simulink model "Demo_SteerableHeadlights_cs"  (R2014b)
settings: Solver=FixedStepDiscrete  SolverMode=SingleTasking  StartTime=0.0  StopTime=45  FixedStep=1/20  RelTol=1e-3
PreLoadFcn:
  | mbxruntime.callbacks.PreLoadFcn(bdroot);
  | check_NUTS_defined;
  | 
  | assignin('base',['model_closed_' bdroot],false);
PostLoadFcn:
  | mbxruntime.callbacks.PostLoadFcn(bdroot);
InitFcn:
  | mbxruntime.callbacks.InitFcn(bdroot);
StartFcn:
  | mbxruntime.callbacks.StartFcn(bdroot);
  | 
  | open_system([bdroot '/BMW_X5_1/Scope: steer angle, preview angle, selected angle']);
StopFcn:
  | mbxruntime.callbacks.StopFcn(bdroot);
model workspace: external: MAT-File .\Demo_SteerableHeadlights_cs_hws.mat (data not in the file)
undefined symbols (not defined in the file or in its folder): mbxruntime, tabledata
undefined symbols (not defined in the file): Demo_SteerableHeadlights_cs_1a268cb91cfaa718, Demo_SteerableHeadlights_cs_a8b5e2ccc8aad9ca, Demo_SteerableHeadlights_cs_BMW_X5_1_Path_pathUniqueID, Demo_SteerableHeadlights_cs_HumanTextured_1_Path_pathUniqueID, SteeringColumn, SteeringWheel, WheelL0, WheelL1, WheelR0, WheelR1
libraries: simulink_extras x15, simulink x2
(part 2 of 5)

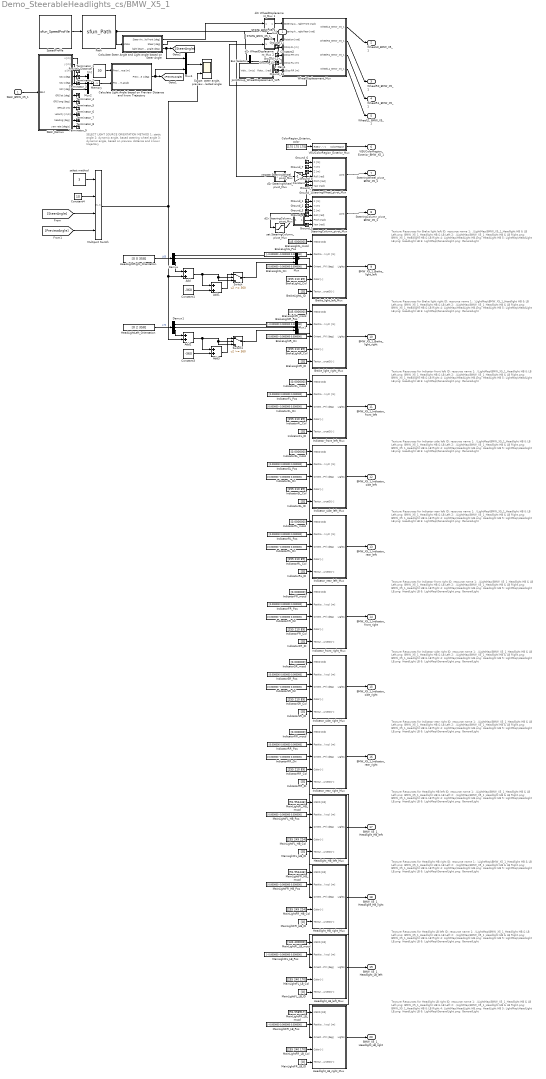
== system Demo_SteerableHeadlights_cs/BMW_X5_1 ==
  note: Texture Resources for Brake light left
      |
      | ID: resource name
      | 1: .\LightMap\BMW_X5_1_Headlight HB & LB Left.png: BMW_X5_1_Headlight HB & LB Left
      | 2: .\LightMap\BMW_X5_1_Headlight HB & LB Right.png: BMW_X5_1_Headlight HB & LB Right
      | 4: LightMap\HeadLight HB.png: HeadLight HB
      | 5: LightMap\HeadLight LB.png: HeadLight LB
      | 6: LightMap\GeneralLight.png: GeneralLight
  note: Texture Resources for Brake light right
      |
      | ID: resource name
      | 1: .\LightMap\BMW_X5_1_Headlight HB & LB Left.png: BMW_X5_1_Headlight HB & LB Left
      | 2: .\LightMap\BMW_X5_1_Headlight HB & LB Right.png: BMW_X5_1_Headlight HB & LB Right
      | 4: LightMap\HeadLight HB.png: HeadLight HB
      | 5: LightMap\HeadLight LB.png: HeadLight LB
      | 6: LightMap\GeneralLight.png: GeneralLight
  note: Texture Resources for Indicator front left
      |
      | ID: resource name
      | 1: .\LightMap\BMW_X5_1_Headlight HB & LB Left.png: BMW_X5_1_Headlight HB & LB Left
      | 2: .\LightMap\BMW_X5_1_Headlight HB & LB Right.png: BMW_X5_1_Headlight HB & LB Right
      | 4: LightMap\HeadLight HB.png: HeadLight HB
      | 5: LightMap\HeadLight LB.png: HeadLight LB
      | 6: LightMap\GeneralLight.png: GeneralLight
  note: Texture Resources for Indicator side left
      |
      | ID: resource name
      | 1: .\LightMap\BMW_X5_1_Headlight HB & LB Left.png: BMW_X5_1_Headlight HB & LB Left
      | 2: .\LightMap\BMW_X5_1_Headlight HB & LB Right.png: BMW_X5_1_Headlight HB & LB Right
      | 4: LightMap\HeadLight HB.png: HeadLight HB
      | 5: LightMap\HeadLight LB.png: HeadLight LB
      | 6: LightMap\GeneralLight.png: GeneralLight
  note: Texture Resources for Indicator rear left
      |
      | ID: resource name
      | 1: .\LightMap\BMW_X5_1_Headlight HB & LB Left.png: BMW_X5_1_Headlight HB & LB Left
      | 2: .\LightMap\BMW_X5_1_Headlight HB & LB Right.png: BMW_X5_1_Headlight HB & LB Right
      | 4: LightMap\HeadLight HB.png: HeadLight HB
      | 5: LightMap\HeadLight LB.png: HeadLight LB
      | 6: LightMap\GeneralLight.png: GeneralLight
  note: Texture Resources for Indicator front right
      |
      | ID: resource name
      | 1: .\LightMap\BMW_X5_1_Headlight HB & LB Left.png: BMW_X5_1_Headlight HB & LB Left
      | 2: .\LightMap\BMW_X5_1_Headlight HB & LB Right.png: BMW_X5_1_Headlight HB & LB Right
      | 4: LightMap\HeadLight HB.png: HeadLight HB
      | 5: LightMap\HeadLight LB.png: HeadLight LB
      | 6: LightMap\GeneralLight.png: GeneralLight
  note: Texture Resources for Indicator side right
      |
      | ID: resource name
      | 1: .\LightMap\BMW_X5_1_Headlight HB & LB Left.png: BMW_X5_1_Headlight HB & LB Left
      | 2: .\LightMap\BMW_X5_1_Headlight HB & LB Right.png: BMW_X5_1_Headlight HB & LB Right
      | 4: LightMap\HeadLight HB.png: HeadLight HB
      | 5: LightMap\HeadLight LB.png: HeadLight LB
      | 6: LightMap\GeneralLight.png: GeneralLight
  note: Texture Resources for Indicator rear right
      |
      | ID: resource name
      | 1: .\LightMap\BMW_X5_1_Headlight HB & LB Left.png: BMW_X5_1_Headlight HB & LB Left
      | 2: .\LightMap\BMW_X5_1_Headlight HB & LB Right.png: BMW_X5_1_Headlight HB & LB Right
      | 4: LightMap\HeadLight HB.png: HeadLight HB
      | 5: LightMap\HeadLight LB.png: HeadLight LB
      | 6: LightMap\GeneralLight.png: GeneralLight
  note: Texture Resources for Headlight HB left
      |
      | ID: resource name
      | 1: .\LightMap\BMW_X5_1_Headlight HB & LB Left.png: BMW_X5_1_Headlight HB & LB Left
      | 2: .\LightMap\BMW_X5_1_Headlight HB & LB Right.png: BMW_X5_1_Headlight HB & LB Right
      | 4: LightMap\HeadLight HB.png: HeadLight HB
      | 5: LightMap\HeadLight LB.png: HeadLight LB
      | 6: LightMap\GeneralLight.png: GeneralLight
  note: Texture Resources for Headlight HB right
      |
      | ID: resource name
      | 1: .\LightMap\BMW_X5_1_Headlight HB & LB Left.png: BMW_X5_1_Headlight HB & LB Left
      | 2: .\LightMap\BMW_X5_1_Headlight HB & LB Right.png: BMW_X5_1_Headlight HB & LB Right
      | 4: LightMap\HeadLight HB.png: HeadLight HB
      | 5: LightMap\HeadLight LB.png: HeadLight LB
      | 6: LightMap\GeneralLight.png: GeneralLight
  note: Texture Resources for Headlight LB left
      |
      | ID: resource name
      | 1: .\LightMap\BMW_X5_1_Headlight HB & LB Left.png: BMW_X5_1_Headlight HB & LB Left
      | 2: .\LightMap\BMW_X5_1_Headlight HB & LB Right.png: BMW_X5_1_Headlight HB & LB Right
      | 4: LightMap\HeadLight HB.png: HeadLight HB
      | 5: LightMap\HeadLight LB.png: HeadLight LB
      | 6: LightMap\GeneralLight.png: GeneralLight
  note: Texture Resources for Headlight LB right
      |
      | ID: resource name
      | 1: .\LightMap\BMW_X5_1_Headlight HB & LB Left.png: BMW_X5_1_Headlight HB & LB Left
      | 2: .\LightMap\BMW_X5_1_Headlight HB & LB Right.png: BMW_X5_1_Headlight HB & LB Right
      | 4: LightMap\HeadLight HB.png: HeadLight HB
      | 5: LightMap\HeadLight LB.png: HeadLight LB
      | 6: LightMap\GeneralLight.png: GeneralLight
  note: SELECT LIGHT SOURCE ORIENTATION METHOD
      | 1: static angle
      | 2: dynamic angle, based steering wheel angle
      | 3: dynamic angle, based on preview distance
      |     and known trajectory
  SELF_BMW_X5_1 : Inport  Tag=inport/SelfPort  OutDataTypeStr=Bus: PRESCAN_SELFSENSORDATA  PortDimensions=1  SampleTime=1/20  BusOutputAsStruct=on
  Add{,1..3} (4 alike) : Sum
  BrakeLightL_Col : Constant  Tag=VisuLightConst  Value=[255 210 89]
  BrakeLightL_ID : Constant  Tag=VisuLightConst  Value=[0]
  BrakeLightL_Ori : Constant  Tag=VisuLightConst  Value=[0.000000 -0.000000 0.000000]
  BrakeLightL_Pos : Constant  Tag=VisuLightConst  Value=[-0.000000 -0.000000 0.000000]
  BrakeLightL_mscd : Constant  Tag=VisuLightConst  Value=[45.000000]
  BrakeLightR_Col : Constant  Tag=VisuLightConst  Value=[255 210 89]
  BrakeLightR_ID : Constant  Tag=VisuLightConst  Value=[0]
  BrakeLightR_Ori : Constant  Tag=VisuLightConst  Value=[0.000000 -0.000000 0.000000]
  BrakeLightR_Pos : Constant  Tag=VisuLightConst  Value=[-0.000000 0.000000 0.000000]
  BrakeLightR_mscd : Constant  Tag=VisuLightConst  Value=[45.000000]
  Brake_light_left_Mux : Subsystem  Tag=mux/ActiveLight  mask(PreScan User Interface: VisuActiveLight){}
      mask help:
      | The VisuActiveLight block provides a way for detailed animation of Light Sources, such as the indicator, brake, fog and main lights of a vehicle, or a light post.
      |
      | For more information, please click Help.
      settings: DeleteFcn=PreScanBlockDeleteFcn;
      mask Help: eval('openHelp(209)')
  Brake_light_right_Mux : Subsystem  Tag=mux/ActiveLight  mask(PreScan User Interface: VisuActiveLight){}
      mask help:
      | The VisuActiveLight block provides a way for detailed animation of Light Sources, such as the indicator, brake, fog and main lights of a vehicle, or a light post.
      |
      | For more information, please click Help.
      settings: DeleteFcn=PreScanBlockDeleteFcn;
      mask Help: eval('openHelp(209)')
  Bus Selector : BusSelector  OutputSignals=VelocityX
  Calculate Light Angle based on Preview Distance and know Trajectory : Subsystem  mask{FileName=PathFollowerSva_1_Synced.mat, TrajOffset=[0 0 0]}
      mask prompts: FileName "Trajectory Name"; TrajOffset "Trajectory Initial Offset x,y,yawangle [m,m,rad]"
      mask init:
      | load(['Trajectories/',FileName])
      | traject=trajectory';
      | 
      | 
      | Traj_x=(traject(:,2)*cos(TrajOffset(3))-traject(:,3)*sin(TrajOffset(3)))+TrajOffset(1);
      | Traj_y=(traject(:,2)*sin(TrajOffset(3))+traject(:,3)*cos(TrajOffset(3)))+TrajOffset(2);
  Calculate Steer Angle and Light angle based on Steer Angle : Subsystem
  ColorRegion_Exterior_color : Constant  Tag=VisuLightConst  Value=[175 175 175]
  Constant : Constant  Value=17
  Constant1 : Constant  Value=-360
  Constant2 : Constant  Value=0
  Constant3 : Constant  Value=-360
  Constant4 : Constant  Value=10
  Demux : Demux  Outputs=3
  Demux1 : Demux  Outputs=3
  Gain4 : Gain  Gain=-1*1.2
  Ground_{1..14} (14 alike) : Ground
  HeadLightLeft_Orientation : Constant  Value=[0 2 358]
  HeadLightRight_Orientation : Constant  Value=[0 0 358]
  Headlight_HB_left_Mux : Subsystem  Tag=mux/ActiveLight  mask(PreScan User Interface: VisuActiveLight){}
      mask help:
      | The VisuActiveLight block provides a way for detailed animation of Light Sources, such as the indicator, brake, fog and main lights of a vehicle, or a light post.
      |
      | For more information, please click Help.
      settings: DeleteFcn=PreScanBlockDeleteFcn;
      mask Help: eval('openHelp(209)')
  Headlight_HB_right_Mux : Subsystem  Tag=mux/ActiveLight  mask(PreScan User Interface: VisuActiveLight){}
      mask help:
      | The VisuActiveLight block provides a way for detailed animation of Light Sources, such as the indicator, brake, fog and main lights of a vehicle, or a light post.
      |
      | For more information, please click Help.
      settings: DeleteFcn=PreScanBlockDeleteFcn;
      mask Help: eval('openHelp(209)')
  Headlight_LB_left_Mux : Subsystem  Tag=mux/ActiveLight  mask(PreScan User Interface: VisuActiveLight){}
      mask help:
      | The VisuActiveLight block provides a way for detailed animation of Light Sources, such as the indicator, brake, fog and main lights of a vehicle, or a light post.
      |
      | For more information, please click Help.
      settings: DeleteFcn=PreScanBlockDeleteFcn;
      mask Help: eval('openHelp(209)')
  Headlight_LB_right_Mux : Subsystem  Tag=mux/ActiveLight  mask(PreScan User Interface: VisuActiveLight){}
      mask help:
      | The VisuActiveLight block provides a way for detailed animation of Light Sources, such as the indicator, brake, fog and main lights of a vehicle, or a light post.
      |
      | For more information, please click Help.
      settings: DeleteFcn=PreScanBlockDeleteFcn;
      mask Help: eval('openHelp(209)')
  IndicatorFL_Col : Constant  Tag=VisuLightConst  Value=[255 210 89]
  IndicatorFL_ID : Constant  Tag=VisuLightConst  Value=[0]
  IndicatorFL_Ori : Constant  Tag=VisuLightConst  Value=[0.000000 -0.000000 0.000000]
  IndicatorFL_Pos : Constant  Tag=VisuLightConst  Value=[0.000000 0.000000 0.000000]
  IndicatorFL_mscd : Constant  Tag=VisuLightConst  Value=[0.000000]
  IndicatorFR_Col : Constant  Tag=VisuLightConst  Value=[255 210 89]
  IndicatorFR_ID : Constant  Tag=VisuLightConst  Value=[0]
  IndicatorFR_Ori : Constant  Tag=VisuLightConst  Value=[0.000000 -0.000000 0.000000]
  IndicatorFR_Pos : Constant  Tag=VisuLightConst  Value=[0.000000 0.000000 0.000000]
  IndicatorFR_mscd : Constant  Tag=VisuLightConst  Value=[0.000000]
  IndicatorRL_Col : Constant  Tag=VisuLightConst  Value=[255 210 89]
  IndicatorRL_ID : Constant  Tag=VisuLightConst  Value=[0]
  IndicatorRL_Ori : Constant  Tag=VisuLightConst  Value=[0.000000 -0.000000 0.000000]
  IndicatorRL_Pos : Constant  Tag=VisuLightConst  Value=[0.000000 0.000000 0.000000]
  IndicatorRL_mscd : Constant  Tag=VisuLightConst  Value=[0.000000]
  IndicatorRR_Col : Constant  Tag=VisuLightConst  Value=[255 210 89]
  IndicatorRR_ID : Constant  Tag=VisuLightConst  Value=[0]
  IndicatorRR_Ori : Constant  Tag=VisuLightConst  Value=[0.000000 -0.000000 0.000000]
  IndicatorRR_Pos : Constant  Tag=VisuLightConst  Value=[0.000000 0.000000 0.000000]
  IndicatorRR_mscd : Constant  Tag=VisuLightConst  Value=[0.000000]
  IndicatorSL_Col : Constant  Tag=VisuLightConst  Value=[255 210 89]
  IndicatorSL_ID : Constant  Tag=VisuLightConst  Value=[0]
  IndicatorSL_Ori : Constant  Tag=VisuLightConst  Value=[0.000000 -0.000000 0.000000]
  IndicatorSL_Pos : Constant  Tag=VisuLightConst  Value=[0.000000 0.000000 0.000000]
  IndicatorSL_mscd : Constant  Tag=VisuLightConst  Value=[0.000000]
  IndicatorSR_Col : Constant  Tag=VisuLightConst  Value=[255 210 89]
  IndicatorSR_ID : Constant  Tag=VisuLightConst  Value=[0]
  IndicatorSR_Ori : Constant  Tag=VisuLightConst  Value=[0.000000 -0.000000 0.000000]
  IndicatorSR_Pos : Constant  Tag=VisuLightConst  Value=[0.000000 0.000000 0.000000]
  IndicatorSR_mscd : Constant  Tag=VisuLightConst  Value=[0.000000]
  Indicator_front_left_Mux : Subsystem  Tag=mux/ActiveLight  mask(PreScan User Interface: VisuActiveLight){}
      mask help:
      | The VisuActiveLight block provides a way for detailed animation of Light Sources, such as the indicator, brake, fog and main lights of a vehicle, or a light post.
      |
      | For more information, please click Help.
      settings: DeleteFcn=PreScanBlockDeleteFcn;
      mask Help: eval('openHelp(209)')
  Indicator_front_right_Mux : Subsystem  Tag=mux/ActiveLight  mask(PreScan User Interface: VisuActiveLight){}
      mask help:
      | The VisuActiveLight block provides a way for detailed animation of Light Sources, such as the indicator, brake, fog and main lights of a vehicle, or a light post.
      |
      | For more information, please click Help.
      settings: DeleteFcn=PreScanBlockDeleteFcn;
      mask Help: eval('openHelp(209)')
  Indicator_rear_left_Mux : Subsystem  Tag=mux/ActiveLight  mask(PreScan User Interface: VisuActiveLight){}
      mask help:
      | The VisuActiveLight block provides a way for detailed animation of Light Sources, such as the indicator, brake, fog and main lights of a vehicle, or a light post.
      |
      | For more information, please click Help.
      settings: DeleteFcn=PreScanBlockDeleteFcn;
      mask Help: eval('openHelp(209)')
  Indicator_rear_right_Mux : Subsystem  Tag=mux/ActiveLight  mask(PreScan User Interface: VisuActiveLight){}
      mask help:
      | The VisuActiveLight block provides a way for detailed animation of Light Sources, such as the indicator, brake, fog and main lights of a vehicle, or a light post.
      |
      | For more information, please click Help.
      settings: DeleteFcn=PreScanBlockDeleteFcn;
      mask Help: eval('openHelp(209)')
  Indicator_side_left_Mux : Subsystem  Tag=mux/ActiveLight  mask(PreScan User Interface: VisuActiveLight){}
      mask help:
      | The VisuActiveLight block provides a way for detailed animation of Light Sources, such as the indicator, brake, fog and main lights of a vehicle, or a light post.
      |
      | For more information, please click Help.
      settings: DeleteFcn=PreScanBlockDeleteFcn;
      mask Help: eval('openHelp(209)')
  Indicator_side_right_Mux : Subsystem  Tag=mux/ActiveLight  mask(PreScan User Interface: VisuActiveLight){}
      mask help:
      | The VisuActiveLight block provides a way for detailed animation of Light Sources, such as the indicator, brake, fog and main lights of a vehicle, or a light post.
      |
      | For more information, please click Help.
      settings: DeleteFcn=PreScanBlockDeleteFcn;
      mask Help: eval('openHelp(209)')
  JointGroup_WheelDisplacement_V2R : Subsystem  Tag=mux/Wheels  mask(PreScan Velocity to Wheel Angle Block:){TimeStep=1/20, TireRadius=0.29}
      mask prompts: TimeStep "Auto Assigned: Time Step [s]"; TireRadius "Tire Radius [m]"
      settings: DeleteFcn=PreScanBlockDeleteFcn;
      mask Display: disp('Velocity\nto\nWheelAngle')
  MainLightFL_HB_Col : Constant  Tag=VisuLightConst  Value=[255 249 224]
  MainLightFL_HB_ID : Constant  Tag=VisuLightConst  Value=[0]
  MainLightFL_HB_Pos : Constant  Tag=VisuLightConst  Value=[0.000000 -0.000000 0.000000]
  MainLightFL_HB_mscd : Constant  Tag=VisuLightConst  Value=[91.954446]
  MainLightFL_LB_Col : Constant  Tag=VisuLightConst  Value=[255 240 170]
  MainLightFL_LB_ID : Constant  Tag=VisuLightConst  Value=[0]
  MainLightFL_LB_Pos : Constant  Tag=VisuLightConst  Value=[-0.000000 -0.000000 0.000000]
  MainLightFL_LB_mscd : Constant  Tag=VisuLightConst  Value=[132.400000]
  MainLightFR_HB_Col : Constant  Tag=VisuLightConst  Value=[255 249 224]
  MainLightFR_HB_ID : Constant  Tag=VisuLightConst  Value=[0]
  MainLightFR_HB_Pos : Constant  Tag=VisuLightConst  Value=[0.000000 -0.000000 0.000000]
  MainLightFR_HB_mscd : Constant  Tag=VisuLightConst  Value=[91.954446]
  MainLightFR_LB_Col : Constant  Tag=VisuLightConst  Value=[255 240 170]
  MainLightFR_LB_ID : Constant  Tag=VisuLightConst  Value=[0]
  MainLightFR_LB_Pos : Constant  Tag=VisuLightConst  Value=[-0.000000 0.000000 0.000000]
  MainLightFR_LB_mscd : Constant  Tag=VisuLightConst  Value=[91.558917]
  Memory : Memory
  Multiport Switch : MultiPortSwitch
  Mux : Mux  Inputs=3
  Mux1 : Mux  Inputs=3
  Mux2 : Mux  Inputs=3
  Mux4 : Mux  Inputs=2
  Path : S-Function  Tag=Path  LoadFcn=load('PrescanMotionData.mat')  FunctionName=sfun_Path  Parameters=uniqueID, pathUniqueID, timestep  EnableBusSupport=off  mask(Path){uniqueID=67, pathUniqueID=Demo_SteerableHeadlights_cs_BMW_X5_1_Path_pathUniqueID, timestep=1/20}
      mask prompts: uniqueID "Object Unique ID"; pathUniqueID "Path Unique ID"; timestep "MATLAB timestep:"
      mask help:
      | The path block outputs the position along a given trajectory.
      |
      | For more information, please click Help.
      mask Help: eval('openHelp(312)')
      mask Display: image(imread('Path.png'))
  Preview Distance [m] : Constant  Value=30
  SELF_Demux : Subsystem  Tag=demux/SelfPort  mask(PreScan Demux Block:){}
      mask help:
      | The SELF port shows (state) information of the actor itself. The outputs are position in the experiment's axis system and the GPS coordinates, and the object's absolute velocity and compass heading.
      |
      | For more information, please click Help.
      settings: DeleteFcn=PreScanBlockDeleteFcn;
      mask Help: eval('openHelp(462)')
      mask Display:
      | port_label('output',1,'x [m]')
      | port_label('output',2,'y [m]')
      | port_label('output',3,'z [m]','texmode','on')
      | port_label('output',4,'Rotx [deg]','texmode','on')
      | port_label('output',5,'Roty [deg]','texmode','on')
      | port_label('output',6,'Rotz [deg]','texmode','on')
      | port_label('output',7,'GPS lat [deg]','texmode','on')
      | port_label('output',8,'GPS long [deg]','texmode','on')
      | port_label('output',9,'GPS alt [m]','texmode','on')
      | port_label('output',10,'Velocity [m/s]')
      | port_label('output',11,'Heading [deg]')
      | port_label('output',12,'Yaw rate [deg/s]')
  STATE_BMW_X5_1_rc : RateTransition  Tag=mux_rc/StatePort  OutPortSampleTimeOpt=Inherit
  "Scope: steer angle, preview angle, selected angle" : Scope  NumInputPorts=2
      settings: TimeRange=45  YMin=-50~-40  YMax=60~45  SaveName=ScopeData2
  SpeedProfile : S-Function  Tag=SpeedProfile  LoadFcn=load('PrescanMotionData.mat')  FunctionName=sfun_SpeedProfile  Parameters=speedProfileUniqueID, timestep  EnableBusSupport=off  mask(SpeedProfile){speedProfileUniqueID=Demo_SteerableHeadlights_cs_1a268cb91cfaa718, timestep=1/20}
      mask prompts: speedProfileUniqueID "Speed Profile Unique ID"; timestep "MATLAB timestep:"
      mask help:
      | The speed profile block outputs the travelled distance, velocities and acceleration along a given path.
      |
      | For more information, please click Help.
      mask Help: eval('openHelp(312)')
      mask Display: image(imread('SpeedProfile.png'))
  SteeringColumn_pivot_Mux : Subsystem  Tag=mux/Joint  mask(PreScan Mux Block){DisplayName=SteeringColumn}
      mask prompts: DisplayName "Display Name"
      mask help:
      | This block simulates a generic joint used for generic models. This joint can be enabled/disabled from the GUI.
      |
      | For more information, please click Help.
      settings: DeleteFcn=PreScanBlockDeleteFcn;
      mask Help: eval('openHelp(254)')
  SteeringWheel_pivot_Mux : Subsystem  Tag=mux/Joint  mask(PreScan Mux Block){DisplayName=SteeringWheel}
      mask prompts: DisplayName "Display Name"
      mask help:
      | This block simulates a generic joint used for generic models. This joint can be enabled/disabled from the GUI.
      |
      | For more information, please click Help.
      settings: DeleteFcn=PreScanBlockDeleteFcn;
      mask Help: eval('openHelp(254)')
  Switch : Switch  Threshold=360
  Switch1 : Switch  Threshold=360
  Terminator_{1..9} (9 alike) : Terminator
  VISUColorRegion_Exterior_Mux : Subsystem  Tag=mux/MuxColorRegion  LoadFcn=load PrescanColorData  mask(PreScan User Interface: VisuTextureColor){}
      mask help:
      | The VisuTextureColor block provides a way to adapt the color of a vehicle.
      |
      | For more information, please click Help.
      settings: DeleteFcn=PreScanBlockDeleteFcn;
      mask Help: eval('openHelp(230)')
  WheelDisplacement_Mux : Subsystem  Tag=mux/JointGroup  mask(JointGroup){}
      mask help:
      | The JointGroup allows to control several Joints in one go, as defined for this particular model.
      | For more information, look in the PreScan manual in the section "Model Preparation Tool" -> "Joint Groups"
      |
      | For more information on the Joints simulink interface, press Help.
      mask Help: eval('openHelp(254)')
  d2r SteeringColumn_pivot_Mux : Subsystem  mask(DegreesToRadians){}
      mask help: SimulinkBlocks:simulink_extras:DegreesToRadians_MD
      mask Help: web([docroot '/simulink/ref_extras/degreestoradians.html'])
      mask Display: disp('D2R')
  d2r SteeringWheel_pivot_Mux : Subsystem  mask(DegreesToRadians){}
      mask help: SimulinkBlocks:simulink_extras:DegreesToRadians_MD
      mask Help: web([docroot '/simulink/ref_extras/degreestoradians.html'])
      mask Display: disp('D2R')
  d2r WheelDisplacement_Mux 1 : Subsystem  mask(DegreesToRadians){}
      mask help: SimulinkBlocks:simulink_extras:DegreesToRadians_MD
      mask Help: web([docroot '/simulink/ref_extras/degreestoradians.html'])
      mask Display: disp('D2R')
  d2r WheelDisplacement_Mux 2 : Subsystem  mask(DegreesToRadians){}
      mask help: SimulinkBlocks:simulink_extras:DegreesToRadians_MD
      mask Help: web([docroot '/simulink/ref_extras/degreestoradians.html'])
      mask Display: disp('D2R')
  negate SteeringWheel_pivot_Mux : Gain  Gain=-1
  sat SteeringColumn_pivot_Mux : Saturate  UpperLimit=30  LowerLimit=-5
  select method : Constant  Value=3
  STATE_BMW_X5_1_bus : Outport  Tag=outport/StatePort  OutDataTypeStr=Bus: PRESCAN_STATEACTUATORDATA  PortDimensions=1  SampleTime=1/20
  WheelL0_BMW_X5_1 : Outport  Tag=outport/JointActuator  Port=2  OutDataTypeStr=Bus: PRESCAN_POSE_DATA  SampleTime=1/20
  WheelR0_BMW_X5_1 : Outport  Tag=outport/JointActuator  Port=3  OutDataTypeStr=Bus: PRESCAN_POSE_DATA  SampleTime=1/20
  WheelR1_BMW_X5_1 : Outport  Tag=outport/JointActuator  Port=4  OutDataTypeStr=Bus: PRESCAN_POSE_DATA  SampleTime=1/20
  WheelL1_BMW_X5_1 : Outport  Tag=outport/JointActuator  Port=5  OutDataTypeStr=Bus: PRESCAN_POSE_DATA  SampleTime=1/20
  VISUColorRegion_Exterior_BMW_X5_1 : Outport  Tag=outport/ColorRegion  Port=6  OutDataTypeStr=Bus: PRESCAN_COLOR_DATA  PortDimensions=1  SampleTime=1/20
  SteeringWheel_pivot_BMW_X5_1 : Outport  Tag=outport/JointActuator  Port=7  OutDataTypeStr=Bus: PRESCAN_POSE_DATA  SampleTime=1/20
  SteeringColumn_pivot_BMW_X5_1 : Outport  Tag=outport/JointActuator  Port=8  OutDataTypeStr=Bus: PRESCAN_POSE_DATA  SampleTime=1/20
  BMW_X5_1_Brake_light_left : Outport  Tag=outport/BrakeLightL  Port=9  OutDataTypeStr=Bus: PRESCAN_VISULIGHTACTUATOR_DATA  SampleTime=1/20
  BMW_X5_1_Brake_light_right : Outport  Tag=outport/BrakeLightR  Port=10  OutDataTypeStr=Bus: PRESCAN_VISULIGHTACTUATOR_DATA  SampleTime=1/20
  BMW_X5_1_Indicator_front_left : Outport  Tag=outport/IndicatorFL  Port=11  OutDataTypeStr=Bus: PRESCAN_VISULIGHTACTUATOR_DATA  SampleTime=1/20
  BMW_X5_1_Indicator_side_left : Outport  Tag=outport/IndicatorSL  Port=12  OutDataTypeStr=Bus: PRESCAN_VISULIGHTACTUATOR_DATA  SampleTime=1/20
  BMW_X5_1_Indicator_rear_left : Outport  Tag=outport/IndicatorRL  Port=13  OutDataTypeStr=Bus: PRESCAN_VISULIGHTACTUATOR_DATA  SampleTime=1/20
  BMW_X5_1_Indicator_front_right : Outport  Tag=outport/IndicatorFR  Port=14  OutDataTypeStr=Bus: PRESCAN_VISULIGHTACTUATOR_DATA  SampleTime=1/20
  BMW_X5_1_Indicator_side_right : Outport  Tag=outport/IndicatorSR  Port=15  OutDataTypeStr=Bus: PRESCAN_VISULIGHTACTUATOR_DATA  SampleTime=1/20
  BMW_X5_1_Indicator_rear_right : Outport  Tag=outport/IndicatorRR  Port=16  OutDataTypeStr=Bus: PRESCAN_VISULIGHTACTUATOR_DATA  SampleTime=1/20
  BMW_X5_1_Headlight_HB_left : Outport  Tag=outport/MainLightFL_HB  Port=17  OutDataTypeStr=Bus: PRESCAN_VISULIGHTACTUATOR_DATA  SampleTime=1/20
  BMW_X5_1_Headlight_HB_right : Outport  Tag=outport/MainLightFR_HB  Port=18  OutDataTypeStr=Bus: PRESCAN_VISULIGHTACTUATOR_DATA  SampleTime=1/20
  BMW_X5_1_Headlight_LB_left : Outport  Tag=outport/MainLightFL_LB  Port=19  OutDataTypeStr=Bus: PRESCAN_VISULIGHTACTUATOR_DATA  SampleTime=1/20
  BMW_X5_1_Headlight_LB_right : Outport  Tag=outport/MainLightFR_LB  Port=20  OutDataTypeStr=Bus: PRESCAN_VISULIGHTACTUATOR_DATA  SampleTime=1/20
  wires:
  Add/1 -> Switch/3, Switch/2, Add1/1
  Switch/1 -> Mux/3
  Demux/1 -> Mux/1
  Demux/2 -> Mux/2
  Demux/3 -> Add/1
  HeadLightRight_Orientation/1 -> Demux/1  "L63"
  Add1/1 -> Switch/1
  Constant1/1 -> Add1/2
  Multiport Switch/1 -> Add2/2, Add/2, "Scope: steer angle, preview angle, selected angle"/2
  Add2/1 -> Switch1/3, Switch1/2, Add3/1
  Switch1/1 -> Mux1/3
  Demux1/1 -> Mux1/1
  Demux1/2 -> Mux1/2
  Demux1/3 -> Add2/1
  HeadLightLeft_Orientation/1 -> Demux1/1  "L70"
  Add3/1 -> Switch1/1
  Constant3/1 -> Add3/2
  Mux4/1 -> "Scope: steer angle, preview angle, selected angle"/1
  Calculate Steer Angle and Light angle based on Steer Angle/1(Steer Angle Front [deg]) -> d2r WheelDisplacement_Mux 1/1(Degrees in)
  Calculate Steer Angle and Light angle based on Steer Angle/2(Steer [deg]) -> d2r SteeringWheel_pivot_Mux/1(Degrees in)
  d2r SteeringWheel_pivot_Mux/1(Radians out) -> negate SteeringWheel_pivot_Mux/1
  Calculate Steer Angle and Light angle based on Steer Angle/3(light beam angle [deg]) -> Mux4/1, [SteerAngle]
  Calculate Light Angle based on Preview Distance and know Trajectory/1(PreviewAngle  [deg]) -> Mux4/2, [PreviewAngle]
  Preview Distance [m]/1 -> Calculate Light Angle based on Preview Distance and know Trajectory/1(Preview Distance [m])
  Memory/1 -> Calculate Light Angle based on Preview Distance and know Trajectory/2(Pos x,y,Y [m,m,grad])
  Mux2/1 -> Memory/1
  select method/1 -> Multiport Switch/1
  Constant4/1 -> Multiport Switch/2
  [SteerAngle] -> Multiport Switch/3
  [PreviewAngle] -> Multiport Switch/4
  Mux/1 -> Headlight_HB_right_Mux/3(Orientation (RPY) [deg]), Headlight_LB_right_Mux/3(Orientation (RPY) [deg])
  Mux1/1 -> Headlight_HB_left_Mux/3(Orientation (RPY) [deg]), Headlight_LB_left_Mux/3(Orientation (RPY) [deg])
  d2r WheelDisplacement_Mux 1/1(Radians out) -> WheelDisplacement_Mux/1(Steering Angle Front [rad])
  negate SteeringWheel_pivot_Mux/1 -> SteeringWheel_pivot_Mux/4(Roll [rad])
  Path/1 -> Calculate Steer Angle and Light angle based on Steer Angle/1(state), Bus Selector/1, STATE_BMW_X5_1_rc/1
  SELF_Demux/1(x [m]) -> Mux2/1
  SELF_Demux/2(y [m]) -> Mux2/2
  SELF_Demux/6(rotz [deg]) -> Mux2/3
  Bus Selector/1 -> Gain4/1
  Gain4/1 -> JointGroup_WheelDisplacement_V2R/1(Velocity [m/s])
  Constant/1 -> sat SteeringColumn_pivot_Mux/1
  sat SteeringColumn_pivot_Mux/1 -> d2r SteeringColumn_pivot_Mux/1(Degrees in)
  d2r SteeringColumn_pivot_Mux/1(Radians out) -> SteeringColumn_pivot_Mux/5(Pitch [rad])
  Constant2/1 -> d2r WheelDisplacement_Mux 2/1(Degrees in)
  d2r WheelDisplacement_Mux 2/1(Radians out) -> WheelDisplacement_Mux/2(Steering Angle Rear [rad])
  STATE_BMW_X5_1_rc/1 -> STATE_BMW_X5_1_bus/1
  SpeedProfile/1 -> Path/1
  SELF_BMW_X5_1/1 -> SELF_Demux/1(SELF)
  WheelDisplacement_Mux/1(WheelL0_BMW_X5_1) -> WheelL0_BMW_X5_1/1
  WheelDisplacement_Mux/2(WheelR0_BMW_X5_1) -> WheelR0_BMW_X5_1/1
  WheelDisplacement_Mux/3(WheelR1_BMW_X5_1) -> WheelR1_BMW_X5_1/1
  WheelDisplacement_Mux/4(WheelL1_BMW_X5_1) -> WheelL1_BMW_X5_1/1
  JointGroup_WheelDisplacement_V2R/1(Rotation [rad]) -> WheelDisplacement_Mux/3(Rotation [rad])
  VISUColorRegion_Exterior_Mux/1(ColorRegion) -> VISUColorRegion_Exterior_BMW_X5_1/1
  ColorRegion_Exterior_color/1 -> VISUColorRegion_Exterior_Mux/1(RGB [-,-,-])
  SteeringWheel_pivot_Mux/1(Joint) -> SteeringWheel_pivot_BMW_X5_1/1
  SteeringColumn_pivot_Mux/1(Joint) -> SteeringColumn_pivot_BMW_X5_1/1
  Brake_light_left_Mux/1(Lights) -> BMW_X5_1_Brake_light_left/1
  BrakeLightL_mscd/1 -> Brake_light_left_Mux/1(MSCD [Cd])
  BrakeLightL_Pos/1 -> Brake_light_left_Mux/2(Position (xyz) [m])
  BrakeLightL_Ori/1 -> Brake_light_left_Mux/3(Orientation (RPY) [deg])
  BrakeLightL_Col/1 -> Brake_light_left_Mux/4(Color [-])
  BrakeLightL_ID/1 -> Brake_light_left_Mux/5(TextureResourceID [-])
  Brake_light_right_Mux/1(Lights) -> BMW_X5_1_Brake_light_right/1
  BrakeLightR_mscd/1 -> Brake_light_right_Mux/1(MSCD [Cd])
  BrakeLightR_Pos/1 -> Brake_light_right_Mux/2(Position (xyz) [m])
  BrakeLightR_Ori/1 -> Brake_light_right_Mux/3(Orientation (RPY) [deg])
  BrakeLightR_Col/1 -> Brake_light_right_Mux/4(Color [-])
  BrakeLightR_ID/1 -> Brake_light_right_Mux/5(TextureResourceID [-])
  Indicator_front_left_Mux/1(Lights) -> BMW_X5_1_Indicator_front_left/1
  IndicatorFL_mscd/1 -> Indicator_front_left_Mux/1(MSCD [Cd])
  IndicatorFL_Pos/1 -> Indicator_front_left_Mux/2(Position (xyz) [m])
  IndicatorFL_Ori/1 -> Indicator_front_left_Mux/3(Orientation (RPY) [deg])
  IndicatorFL_Col/1 -> Indicator_front_left_Mux/4(Color [-])
  IndicatorFL_ID/1 -> Indicator_front_left_Mux/5(TextureResourceID [-])
  Indicator_side_left_Mux/1(Lights) -> BMW_X5_1_Indicator_side_left/1
  IndicatorSL_mscd/1 -> Indicator_side_left_Mux/1(MSCD [Cd])
  IndicatorSL_Pos/1 -> Indicator_side_left_Mux/2(Position (xyz) [m])
  IndicatorSL_Ori/1 -> Indicator_side_left_Mux/3(Orientation (RPY) [deg])
  IndicatorSL_Col/1 -> Indicator_side_left_Mux/4(Color [-])
  IndicatorSL_ID/1 -> Indicator_side_left_Mux/5(TextureResourceID [-])
  Indicator_rear_left_Mux/1(Lights) -> BMW_X5_1_Indicator_rear_left/1
  IndicatorRL_mscd/1 -> Indicator_rear_left_Mux/1(MSCD [Cd])
  IndicatorRL_Pos/1 -> Indicator_rear_left_Mux/2(Position (xyz) [m])
  IndicatorRL_Ori/1 -> Indicator_rear_left_Mux/3(Orientation (RPY) [deg])
  IndicatorRL_Col/1 -> Indicator_rear_left_Mux/4(Color [-])
  IndicatorRL_ID/1 -> Indicator_rear_left_Mux/5(TextureResourceID [-])
  Indicator_front_right_Mux/1(Lights) -> BMW_X5_1_Indicator_front_right/1
  IndicatorFR_mscd/1 -> Indicator_front_right_Mux/1(MSCD [Cd])
  IndicatorFR_Pos/1 -> Indicator_front_right_Mux/2(Position (xyz) [m])
  IndicatorFR_Ori/1 -> Indicator_front_right_Mux/3(Orientation (RPY) [deg])
  IndicatorFR_Col/1 -> Indicator_front_right_Mux/4(Color [-])
  IndicatorFR_ID/1 -> Indicator_front_right_Mux/5(TextureResourceID [-])
  Indicator_side_right_Mux/1(Lights) -> BMW_X5_1_Indicator_side_right/1
  IndicatorSR_mscd/1 -> Indicator_side_right_Mux/1(MSCD [Cd])
  IndicatorSR_Pos/1 -> Indicator_side_right_Mux/2(Position (xyz) [m])
  IndicatorSR_Ori/1 -> Indicator_side_right_Mux/3(Orientation (RPY) [deg])
  IndicatorSR_Col/1 -> Indicator_side_right_Mux/4(Color [-])
  IndicatorSR_ID/1 -> Indicator_side_right_Mux/5(TextureResourceID [-])
  Indicator_rear_right_Mux/1(Lights) -> BMW_X5_1_Indicator_rear_right/1
  IndicatorRR_mscd/1 -> Indicator_rear_right_Mux/1(MSCD [Cd])
  IndicatorRR_Pos/1 -> Indicator_rear_right_Mux/2(Position (xyz) [m])
  IndicatorRR_Ori/1 -> Indicator_rear_right_Mux/3(Orientation (RPY) [deg])
  IndicatorRR_Col/1 -> Indicator_rear_right_Mux/4(Color [-])
  IndicatorRR_ID/1 -> Indicator_rear_right_Mux/5(TextureResourceID [-])
  Headlight_HB_left_Mux/1(Lights) -> BMW_X5_1_Headlight_HB_left/1
  MainLightFL_HB_mscd/1 -> Headlight_HB_left_Mux/1(MSCD [Cd])
  MainLightFL_HB_Pos/1 -> Headlight_HB_left_Mux/2(Position (xyz) [m])
  MainLightFL_HB_Col/1 -> Headlight_HB_left_Mux/4(Color [-])
  MainLightFL_HB_ID/1 -> Headlight_HB_left_Mux/5(TextureResourceID [-])
  Headlight_HB_right_Mux/1(Lights) -> BMW_X5_1_Headlight_HB_right/1
  MainLightFR_HB_mscd/1 -> Headlight_HB_right_Mux/1(MSCD [Cd])
  MainLightFR_HB_Pos/1 -> Headlight_HB_right_Mux/2(Position (xyz) [m])
  MainLightFR_HB_Col/1 -> Headlight_HB_right_Mux/4(Color [-])
  MainLightFR_HB_ID/1 -> Headlight_HB_right_Mux/5(TextureResourceID [-])
  Headlight_LB_left_Mux/1(Lights) -> BMW_X5_1_Headlight_LB_left/1
  MainLightFL_LB_mscd/1 -> Headlight_LB_left_Mux/1(MSCD [Cd])
  MainLightFL_LB_Pos/1 -> Headlight_LB_left_Mux/2(Position (xyz) [m])
  MainLightFL_LB_Col/1 -> Headlight_LB_left_Mux/4(Color [-])
  MainLightFL_LB_ID/1 -> Headlight_LB_left_Mux/5(TextureResourceID [-])
  Headlight_LB_right_Mux/1(Lights) -> BMW_X5_1_Headlight_LB_right/1
  MainLightFR_LB_mscd/1 -> Headlight_LB_right_Mux/1(MSCD [Cd])
  MainLightFR_LB_Pos/1 -> Headlight_LB_right_Mux/2(Position (xyz) [m])
  MainLightFR_LB_Col/1 -> Headlight_LB_right_Mux/4(Color [-])
  MainLightFR_LB_ID/1 -> Headlight_LB_right_Mux/5(TextureResourceID [-])
  SELF_Demux/3(z [m]) -> Terminator_1/1
  SELF_Demux/4(rotx [deg]) -> Terminator_2/1
  SELF_Demux/5(roty [deg]) -> Terminator_3/1
  SELF_Demux/7(GPS lat [deg]) -> Terminator_4/1
  SELF_Demux/8(GPS long [deg]) -> Terminator_5/1
  SELF_Demux/9(GPS alt [m]) -> Terminator_6/1
  SELF_Demux/10(velocity [m/s]) -> Terminator_7/1
  SELF_Demux/11(heading [deg]) -> Terminator_8/1
  SELF_Demux/12(yaw rate [deg/s]) -> Terminator_9/1
  Ground_1/1 -> SteeringColumn_pivot_Mux/1(X [m])
  Ground_2/1 -> SteeringColumn_pivot_Mux/2(Y [m])
  Ground_3/1 -> SteeringColumn_pivot_Mux/3(Z [m])
  Ground_4/1 -> SteeringColumn_pivot_Mux/4(Roll [rad])
  Ground_5/1 -> SteeringColumn_pivot_Mux/6(Yaw [rad])
  Ground_6/1 -> SteeringWheel_pivot_Mux/1(X [m])
  Ground_7/1 -> SteeringWheel_pivot_Mux/2(Y [m])
  Ground_8/1 -> SteeringWheel_pivot_Mux/3(Z [m])
  Ground_9/1 -> SteeringWheel_pivot_Mux/5(Pitch [rad])
  Ground_10/1 -> SteeringWheel_pivot_Mux/6(Yaw [rad])
  Ground_11/1 -> WheelDisplacement_Mux/4(zDisp FL [m])
  Ground_12/1 -> WheelDisplacement_Mux/5(zDisp FR [m])
  Ground_13/1 -> WheelDisplacement_Mux/6(zDisp RL [m])
  Ground_14/1 -> WheelDisplacement_Mux/7(zDisp RR [m])

== system Demo_SteerableHeadlights_cs/BMW_X5_1_Brake_light_left ==
  BMW_X5_1_Brake_light_left : Inport  Tag=inport/BrakeLightL  OutDataTypeStr=Bus: PRESCAN_VISULIGHTACTUATOR_DATA  SampleTime=1/20  BusOutputAsStruct=on
  Actuator : S-Function  FunctionName=sfun_VisuLightActuator  Parameters=mbxruntime.parameters.convert(UniqueID), mbxruntime.parameters.convert(LightName), mbxruntime.parameters.convert(PivotName), mbxruntime.parameters.convert(TextureResources), mbxruntime.parameters.convert(ColorsObjectName), mbxruntime.parameters.convert(MeshOnColor), mbxruntime.parameters.convert(MeshOffColor),tabledata, TimeStep  EnableBusSupport=off  mask(PreScan Sink Block: VisuActiveLight){UniqueID=67, LightName=BMW_X5_1.LightActuator_0_BrakeLightL_ActiveLight, PivotName=BMW_X5_1.BrakeLightL_pivot, TextureResources={ '1' '.\LightMap\BMW_X5_1_Headlight HB & LB Left.png' '2' '.\LightMap\BMW_X5_1_Headlight HB & LB Right.png' '4' 'LightMap\HeadLight HB.png' '5' 'LightMap\HeadLight LB.png' '6' 'LightMap\GeneralLight.png'}, ColorsObjectName=BMW_X5_1.BrakeLightL, MeshOnColor=[255    0    0  255  255    0    0  255  102  102  102  255  510  420  178  255], MeshOffColor=[255    0    0  255  255    0    0  255  102  102  102  255    0    0    0  255], TimeStep=1/20}
      mask prompts: UniqueID "Parent Unique Identifier"; LightName "Light"; PivotName "Pivot"; TextureResources "Texture Resources"; ColorsObjectName "Light Fixture Color Object"; MeshOnColor "Light Fixture On Color"; MeshOffColor "Light Fixture Off Color"; TimeStep "Simulink time step"
      mask help:
      | The VisuActiveLight block provides a way for detailed animation of Light Sources, such as the indicator, brake, fog and main lights of a vehicle, or a light post.
      |
      | For more information, please click Help.
      mask init:
      | [tabledata] = mbxruntime.parameters.table(UniqueID,LightName,PivotName,TextureResources,ColorsObjectName,MeshOnColor,MeshOffColor);
      mask Help: eval('openHelp(209)')
      mask Display: image(imread('HeadLight.png'))
  wires:
  BMW_X5_1_Brake_light_left/1 -> Actuator/1

== system Demo_SteerableHeadlights_cs/BMW_X5_1_Brake_light_right ==
  BMW_X5_1_Brake_light_right : Inport  Tag=inport/BrakeLightR  OutDataTypeStr=Bus: PRESCAN_VISULIGHTACTUATOR_DATA  SampleTime=1/20  BusOutputAsStruct=on
  Actuator : S-Function  FunctionName=sfun_VisuLightActuator  Parameters=mbxruntime.parameters.convert(UniqueID), mbxruntime.parameters.convert(LightName), mbxruntime.parameters.convert(PivotName), mbxruntime.parameters.convert(TextureResources), mbxruntime.parameters.convert(ColorsObjectName), mbxruntime.parameters.convert(MeshOnColor), mbxruntime.parameters.convert(MeshOffColor),tabledata, TimeStep  EnableBusSupport=off  mask(PreScan Sink Block: VisuActiveLight){UniqueID=67, LightName=BMW_X5_1.LightActuator_1_BrakeLightR_ActiveLight, PivotName=BMW_X5_1.BrakeLightR_pivot, TextureResources={ '1' '.\LightMap\BMW_X5_1_Headlight HB & LB Left.png' '2' '.\LightMap\BMW_X5_1_Headlight HB & LB Right.png' '4' 'LightMap\HeadLight HB.png' '5' 'LightMap\HeadLight LB.png' '6' 'LightMap\GeneralLight.png'}, ColorsObjectName=BMW_X5_1.BrakeLightR, MeshOnColor=[255    0    0  255  255    0    0  255  102  102  102  255  510  420  178  255], MeshOffColor=[255    0    0  255  255    0    0  255  102  102  102  255    0    0    0  255], TimeStep=1/20}
      mask prompts: UniqueID "Parent Unique Identifier"; LightName "Light"; PivotName "Pivot"; TextureResources "Texture Resources"; ColorsObjectName "Light Fixture Color Object"; MeshOnColor "Light Fixture On Color"; MeshOffColor "Light Fixture Off Color"; TimeStep "Simulink time step"
      mask help:
      | The VisuActiveLight block provides a way for detailed animation of Light Sources, such as the indicator, brake, fog and main lights of a vehicle, or a light post.
      |
      | For more information, please click Help.
      mask init:
      | [tabledata] = mbxruntime.parameters.table(UniqueID,LightName,PivotName,TextureResources,ColorsObjectName,MeshOnColor,MeshOffColor);
      mask Help: eval('openHelp(209)')
      mask Display: image(imread('HeadLight.png'))
  wires:
  BMW_X5_1_Brake_light_right/1 -> Actuator/1

== system Demo_SteerableHeadlights_cs/BMW_X5_1_Headlight_HB_left ==
  BMW_X5_1_Headlight_HB_left : Inport  Tag=inport/MainLightFL_HB  OutDataTypeStr=Bus: PRESCAN_VISULIGHTACTUATOR_DATA  SampleTime=1/20  BusOutputAsStruct=on
  Actuator : S-Function  FunctionName=sfun_VisuLightActuator  Parameters=mbxruntime.parameters.convert(UniqueID), mbxruntime.parameters.convert(LightName), mbxruntime.parameters.convert(PivotName), mbxruntime.parameters.convert(TextureResources), mbxruntime.parameters.convert(ColorsObjectName), mbxruntime.parameters.convert(MeshOnColor), mbxruntime.parameters.convert(MeshOffColor),tabledata, TimeStep  EnableBusSupport=off  mask(PreScan Sink Block: VisuActiveLight){UniqueID=67, LightName=BMW_X5_1.LightActuator_11_MainLightFL_HB_ActiveLight, PivotName=BMW_X5_1.MainLightFL_HB_pivot, TextureResources={ '1' '.\LightMap\BMW_X5_1_Headlight HB & LB Left.png' '2' '.\LightMap\BMW_X5_1_Headlight HB & LB Right.png' '4' 'LightMap\HeadLight HB.png' '5' 'LightMap\HeadLight LB.png' '6' 'LightMap\GeneralLight.png'}, ColorsObjectName=BMW_X5_1.MainLightFL_HB, MeshOnColor=[255  255  255    0  255  255  255    0  102  102  102  255  510  498  448  255], MeshOffColor=[255  255  255    0  255  255  255    0  102  102  102  255    0    0    0  255], TimeStep=1/20}
      mask prompts: UniqueID "Parent Unique Identifier"; LightName "Light"; PivotName "Pivot"; TextureResources "Texture Resources"; ColorsObjectName "Light Fixture Color Object"; MeshOnColor "Light Fixture On Color"; MeshOffColor "Light Fixture Off Color"; TimeStep "Simulink time step"
      mask help:
      | The VisuActiveLight block provides a way for detailed animation of Light Sources, such as the indicator, brake, fog and main lights of a vehicle, or a light post.
      |
      | For more information, please click Help.
      mask init:
      | [tabledata] = mbxruntime.parameters.table(UniqueID,LightName,PivotName,TextureResources,ColorsObjectName,MeshOnColor,MeshOffColor);
      mask Help: eval('openHelp(209)')
      mask Display: image(imread('HeadLight.png'))
  wires:
  BMW_X5_1_Headlight_HB_left/1 -> Actuator/1

== system Demo_SteerableHeadlights_cs/BMW_X5_1_Headlight_HB_right ==
  BMW_X5_1_Headlight_HB_right : Inport  Tag=inport/MainLightFR_HB  OutDataTypeStr=Bus: PRESCAN_VISULIGHTACTUATOR_DATA  SampleTime=1/20  BusOutputAsStruct=on
  Actuator : S-Function  FunctionName=sfun_VisuLightActuator  Parameters=mbxruntime.parameters.convert(UniqueID), mbxruntime.parameters.convert(LightName), mbxruntime.parameters.convert(PivotName), mbxruntime.parameters.convert(TextureResources), mbxruntime.parameters.convert(ColorsObjectName), mbxruntime.parameters.convert(MeshOnColor), mbxruntime.parameters.convert(MeshOffColor),tabledata, TimeStep  EnableBusSupport=off  mask(PreScan Sink Block: VisuActiveLight){UniqueID=67, LightName=BMW_X5_1.LightActuator_12_MainLightFR_HB_ActiveLight, PivotName=BMW_X5_1.MainLightFR_HB_pivot, TextureResources={ '1' '.\LightMap\BMW_X5_1_Headlight HB & LB Left.png' '2' '.\LightMap\BMW_X5_1_Headlight HB & LB Right.png' '4' 'LightMap\HeadLight HB.png' '5' 'LightMap\HeadLight LB.png' '6' 'LightMap\GeneralLight.png'}, ColorsObjectName=BMW_X5_1.MainLightFR_HB, MeshOnColor=[255  255  255    0  255  255  255    0  102  102  102  255  510  498  448  255], MeshOffColor=[255  255  255    0  255  255  255    0  102  102  102  255    0    0    0  255], TimeStep=1/20}
      mask prompts: UniqueID "Parent Unique Identifier"; LightName "Light"; PivotName "Pivot"; TextureResources "Texture Resources"; ColorsObjectName "Light Fixture Color Object"; MeshOnColor "Light Fixture On Color"; MeshOffColor "Light Fixture Off Color"; TimeStep "Simulink time step"
      mask help:
      | The VisuActiveLight block provides a way for detailed animation of Light Sources, such as the indicator, brake, fog and main lights of a vehicle, or a light post.
      |
      | For more information, please click Help.
      mask init:
      | [tabledata] = mbxruntime.parameters.table(UniqueID,LightName,PivotName,TextureResources,ColorsObjectName,MeshOnColor,MeshOffColor);
      mask Help: eval('openHelp(209)')
      mask Display: image(imread('HeadLight.png'))
  wires:
  BMW_X5_1_Headlight_HB_right/1 -> Actuator/1

== system Demo_SteerableHeadlights_cs/BMW_X5_1_Headlight_LB_left ==
  BMW_X5_1_Headlight_LB_left : Inport  Tag=inport/MainLightFL_LB  OutDataTypeStr=Bus: PRESCAN_VISULIGHTACTUATOR_DATA  SampleTime=1/20  BusOutputAsStruct=on
  Actuator : S-Function  FunctionName=sfun_VisuLightActuator  Parameters=mbxruntime.parameters.convert(UniqueID), mbxruntime.parameters.convert(LightName), mbxruntime.parameters.convert(PivotName), mbxruntime.parameters.convert(TextureResources), mbxruntime.parameters.convert(ColorsObjectName), mbxruntime.parameters.convert(MeshOnColor), mbxruntime.parameters.convert(MeshOffColor),tabledata, TimeStep  EnableBusSupport=off  mask(PreScan Sink Block: VisuActiveLight){UniqueID=67, LightName=BMW_X5_1.LightActuator_13_MainLightFL_LB_ActiveLight, PivotName=BMW_X5_1.MainLightFL_LB_pivot, TextureResources={ '1' '.\LightMap\BMW_X5_1_Headlight HB & LB Left.png' '2' '.\LightMap\BMW_X5_1_Headlight HB & LB Right.png' '4' 'LightMap\HeadLight HB.png' '5' 'LightMap\HeadLight LB.png' '6' 'LightMap\GeneralLight.png'}, ColorsObjectName=BMW_X5_1.MainLightFL_LB, MeshOnColor=[255  255  255    0  255  255  255    0  102  102  102  255  510  480  340  255], MeshOffColor=[255  255  255    0  255  255  255    0  102  102  102  255    0    0    0  255], TimeStep=1/20}
      mask prompts: UniqueID "Parent Unique Identifier"; LightName "Light"; PivotName "Pivot"; TextureResources "Texture Resources"; ColorsObjectName "Light Fixture Color Object"; MeshOnColor "Light Fixture On Color"; MeshOffColor "Light Fixture Off Color"; TimeStep "Simulink time step"
      mask help:
      | The VisuActiveLight block provides a way for detailed animation of Light Sources, such as the indicator, brake, fog and main lights of a vehicle, or a light post.
      |
      | For more information, please click Help.
      mask init:
      | [tabledata] = mbxruntime.parameters.table(UniqueID,LightName,PivotName,TextureResources,ColorsObjectName,MeshOnColor,MeshOffColor);
      mask Help: eval('openHelp(209)')
      mask Display: image(imread('HeadLight.png'))
  wires:
  BMW_X5_1_Headlight_LB_left/1 -> Actuator/1

== system Demo_SteerableHeadlights_cs/BMW_X5_1_Headlight_LB_right ==
  BMW_X5_1_Headlight_LB_right : Inport  Tag=inport/MainLightFR_LB  OutDataTypeStr=Bus: PRESCAN_VISULIGHTACTUATOR_DATA  SampleTime=1/20  BusOutputAsStruct=on
  Actuator : S-Function  FunctionName=sfun_VisuLightActuator  Parameters=mbxruntime.parameters.convert(UniqueID), mbxruntime.parameters.convert(LightName), mbxruntime.parameters.convert(PivotName), mbxruntime.parameters.convert(TextureResources), mbxruntime.parameters.convert(ColorsObjectName), mbxruntime.parameters.convert(MeshOnColor), mbxruntime.parameters.convert(MeshOffColor),tabledata, TimeStep  EnableBusSupport=off  mask(PreScan Sink Block: VisuActiveLight){UniqueID=67, LightName=BMW_X5_1.LightActuator_14_MainLightFR_LB_ActiveLight, PivotName=BMW_X5_1.MainLightFR_LB_pivot, TextureResources={ '1' '.\LightMap\BMW_X5_1_Headlight HB & LB Left.png' '2' '.\LightMap\BMW_X5_1_Headlight HB & LB Right.png' '4' 'LightMap\HeadLight HB.png' '5' 'LightMap\HeadLight LB.png' '6' 'LightMap\GeneralLight.png'}, ColorsObjectName=BMW_X5_1.MainLightFR_LB, MeshOnColor=[255  255  255    0  255  255  255    0  102  102  102  255  510  480  340  255], MeshOffColor=[255  255  255    0  255  255  255    0  102  102  102  255    0    0    0  255], TimeStep=1/20}
      mask prompts: UniqueID "Parent Unique Identifier"; LightName "Light"; PivotName "Pivot"; TextureResources "Texture Resources"; ColorsObjectName "Light Fixture Color Object"; MeshOnColor "Light Fixture On Color"; MeshOffColor "Light Fixture Off Color"; TimeStep "Simulink time step"
      mask help:
      | The VisuActiveLight block provides a way for detailed animation of Light Sources, such as the indicator, brake, fog and main lights of a vehicle, or a light post.
      |
      | For more information, please click Help.
      mask init:
      | [tabledata] = mbxruntime.parameters.table(UniqueID,LightName,PivotName,TextureResources,ColorsObjectName,MeshOnColor,MeshOffColor);
      mask Help: eval('openHelp(209)')
      mask Display: image(imread('HeadLight.png'))
  wires:
  BMW_X5_1_Headlight_LB_right/1 -> Actuator/1

== system Demo_SteerableHeadlights_cs/BMW_X5_1_Indicator_front_left ==
  BMW_X5_1_Indicator_front_left : Inport  Tag=inport/IndicatorFL  OutDataTypeStr=Bus: PRESCAN_VISULIGHTACTUATOR_DATA  SampleTime=1/20  BusOutputAsStruct=on
  Actuator : S-Function  FunctionName=sfun_VisuLightActuator  Parameters=mbxruntime.parameters.convert(UniqueID), mbxruntime.parameters.convert(LightName), mbxruntime.parameters.convert(PivotName), mbxruntime.parameters.convert(TextureResources), mbxruntime.parameters.convert(ColorsObjectName), mbxruntime.parameters.convert(MeshOnColor), mbxruntime.parameters.convert(MeshOffColor),tabledata, TimeStep  EnableBusSupport=off  mask(PreScan Sink Block: VisuActiveLight){UniqueID=67, LightName=BMW_X5_1.LightActuator_5_IndicatorFL_ActiveLight, PivotName=BMW_X5_1.IndicatorFL_pivot, TextureResources={ '1' '.\LightMap\BMW_X5_1_Headlight HB & LB Left.png' '2' '.\LightMap\BMW_X5_1_Headlight HB & LB Right.png' '4' 'LightMap\HeadLight HB.png' '5' 'LightMap\HeadLight LB.png' '6' 'LightMap\GeneralLight.png'}, ColorsObjectName=BMW_X5_1.IndicatorFL, MeshOnColor=[255  165    0    0  255  165    0    0  102  102  102  255  510  420  178  255], MeshOffColor=[255  165    0    0  255  165    0    0  102  102  102  255    0    0    0  255], TimeStep=1/20}
      mask prompts: UniqueID "Parent Unique Identifier"; LightName "Light"; PivotName "Pivot"; TextureResources "Texture Resources"; ColorsObjectName "Light Fixture Color Object"; MeshOnColor "Light Fixture On Color"; MeshOffColor "Light Fixture Off Color"; TimeStep "Simulink time step"
      mask help:
      | The VisuActiveLight block provides a way for detailed animation of Light Sources, such as the indicator, brake, fog and main lights of a vehicle, or a light post.
      |
      | For more information, please click Help.
      mask init:
      | [tabledata] = mbxruntime.parameters.table(UniqueID,LightName,PivotName,TextureResources,ColorsObjectName,MeshOnColor,MeshOffColor);
      mask Help: eval('openHelp(209)')
      mask Display: image(imread('HeadLight.png'))
  wires:
  BMW_X5_1_Indicator_front_left/1 -> Actuator/1
